simulink model "tp2"  (R2013a)
settings: Solver=ode45  StartTime=0.0  StopTime=0.1  RelTol=1e-3
libraries: powerlib x15, simulink x1
settings Model: Creator=DELL  LastModifiedBy=DELL

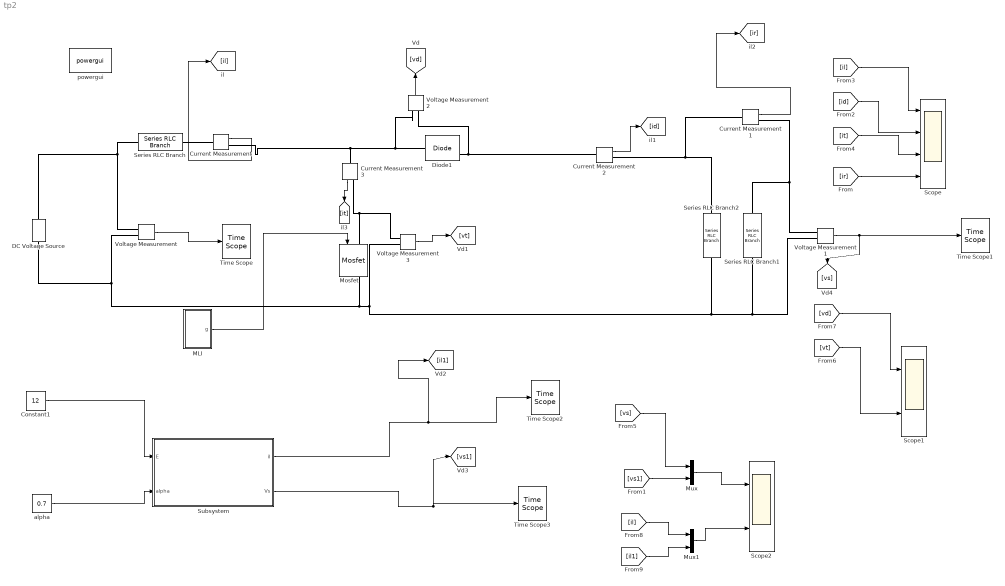
== system tp2 ==
  Constant1 : Constant  Value=12
  Current Measurement{,1..3} (4 alike) : powerlib/Measurements/Current Measurement  PhasorSimulation=off  OutputType=Complex  PSBequivalent=0
  DC Voltage Source : powerlib/Electrical Sources/DC Voltage Source  Amplitude=12  Measurements=Voltage
  Diode1 : powerlib/Power Electronics/Diode  Ron=0.001  Lon=0  Vf=0.8  IC=0  UseSnubber=off  Rs=500  Cs=0  Measurements=on
  "MLI " : Subsystem
  Mosfet : powerlib/Power Electronics/Mosfet  Ron=0.1  Lon=0  Rd=0.01  Vfd=0  IC=0  Rs=1e5  Cs=inf  Measurements=on
  Mux : Mux  Inputs=2
  Mux1 : Mux  Inputs=2
  Scope : Scope  NumInputPorts=4
      settings: YMin=-5~-5~-5~-5  YMax=5~5~5~5
  Scope1 : Scope  NumInputPorts=2
      settings: YMin=-5~-5  YMax=5~5
  Scope2 : Scope  NumInputPorts=2
      settings: YMin=-5~-5  YMax=5~5  SaveName=ScopeData2
  Series RLC Branch : powerlib/Elements/Series RLC Branch  LConnTagsString=__new0  RConnTagsString=__new0  BranchType=L  Resistance=1  Inductance=76.8e-6  SetiL0=off  InitialCurrent=0  Capacitance=1e-6  Setx0=off  InitialVoltage=0  Measurements=None
  Series RLC Branch1 : powerlib/Elements/Series RLC Branch  LConnTagsString=__new0  RConnTagsString=__new0  BranchType=R  Resistance=4  Inductance=1e-3  SetiL0=off  InitialCurrent=0  Capacitance=1e-6  Setx0=off  InitialVoltage=0  Measurements=None
  Series RLC Branch2 : powerlib/Elements/Series RLC Branch  LConnTagsString=__new0  RConnTagsString=__new0  BranchType=C  Resistance=1  Inductance=1e-3  SetiL0=off  InitialCurrent=0  Capacitance=400e-6  Setx0=off  InitialVoltage=0  Measurements=None
  Subsystem : Subsystem
  Time Scope{,1..3} (4 alike) : TimeScope  DefaultConfigurationName=spbscopes.TimeScopeBlockCfg
      settings: CopyFcn=scopeextensions.ScopeBlock.callback(gcbh, 'onBlockCopy', gcbh);  DeleteFcn=scopeextensions.ScopeBlock.callback(gcbh, 'onBlockDelete');  PreSaveFcn=scopeextensions.ScopeBlock.callback(gcbh, 'onModelSave');  NameChangeFcn=scopeextensions.ScopeBlock.callback(gcbh, 'onBlockRename');  CloseFcn=scopeextensions.ScopeBlock.callback(gcbh, 'onBlockClose');  PreDeleteFcn=scopeextensions.ScopeBlock.callback(gcbh, 'onBlockPreDelete');
  Voltage Measurement{,1..3} (4 alike) : powerlib/Measurements/Voltage Measurement  PhasorSimulation=off  OutputType=Complex  PSBequivalent=0
  "alpha " : Constant  Value=0.7
  powergui : powerlib/powergui  Priority=1  SimulationMode=Continuous  SolverType=Tustin  SampleTime=50e-6  frequency=60  SPID=off  DisableSnubberDevices=off  DisableRonSwitches=off  DisableVfSwitches=off  SwTol=0  Interpol=off  DisplayEquations=off  frequencyindice=0  Pbase=100e6  ErrMax=1e-4  Iterations=50  UnitsV=kV  UnitsW=MW  FunctionMessages=off  echomessages=off  HookPort=off  EnableUseOfTLC=off  x0status=blocks  RestoreLinks=warning  ResistiveCurrentMeasurement=off  Frange=[0:2:500]  Ylog=off  Xlog=on  ShowGrid=off  save=off  variable=ZData  ZoomFFT=off  StartTime=0.0  cycles=1  DisplayStyle=1  fundamental=60  FreqAxis=off  MaxFrequency=1000  frequencyindicesteady=1  RmsSteady=1  display=off  Ts=0  methode=off
  wires:
  Voltage Measurement1/1 -> [vs], Time Scope1/1
  Voltage Measurement/1 -> Time Scope/1
  "MLI "/1(g) -> Mosfet/1
  Current Measurement/1 -> [il]
  Voltage Measurement2/1 -> [vd]
  Voltage Measurement3/1 -> [vt]
  [il] -> Scope/1
  [id] -> Scope/2
  [ir] -> Scope/4
  Current Measurement2/1 -> [id]
  Current Measurement1/1 -> [ir]
  [it] -> Scope/3
  Current Measurement3/1 -> [it]
  [vd] -> Scope1/1
  [vt] -> Scope1/2
  Subsystem/1(il) -> [il1], Time Scope2/1
  Constant1/1 -> Subsystem/1(E)
  "alpha "/1 -> Subsystem/2("alpha ")
  Mux/1 -> Scope2/1
  Mux1/1 -> Scope2/2
  Subsystem/2(Vs) -> [vs1], Time Scope3/1
  [vs] -> Mux/1
  [vs1] -> Mux/2
  [il] -> Mux1/1
  [il1] -> Mux1/2
  connections:
  DC Voltage Source/RConn1 -- Voltage Measurement/LConn1 -- Series RLC Branch/LConn1
  DC Voltage Source/LConn1 -- Voltage Measurement/LConn2 -- Mosfet/RConn1 -- Voltage Measurement3/LConn2 -- Series RLC Branch2/RConn1 -- Series RLC Branch1/RConn1 -- Voltage Measurement1/LConn2
  Current Measurement/RConn1 -- Voltage Measurement2/LConn1 -- Diode1/LConn1 -- Current Measurement3/LConn1
  Voltage Measurement2/LConn2 -- Current Measurement2/LConn1 -- Diode1/RConn1
  Series RLC Branch/RConn1 -- Current Measurement/LConn1
  Series RLC Branch1/LConn1 -- Current Measurement1/RConn1 -- Voltage Measurement1/LConn1
  Current Measurement2/RConn1 -- Current Measurement1/LConn1 -- Series RLC Branch2/LConn1
  Voltage Measurement3/LConn1 -- Current Measurement3/RConn1 -- Mosfet/LConn1

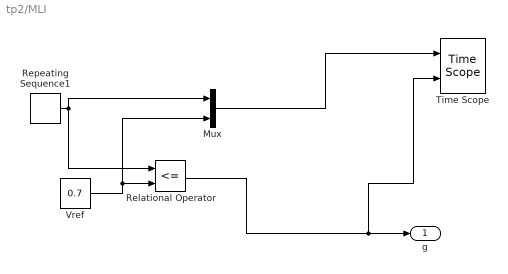
== system tp2/MLI  ==
  Mux : Mux  Inputs=2
  Relational Operator : RelationalOperator  Operator=<=  OutDataTypeStr=boolean
  Repeating Sequence1 : simulink/Sources/Repeating Sequence  rep_seq_t=[0 (1/20000) (1/10000)]  rep_seq_y=[0 1 0]
  Time Scope : TimeScope  NumInputPorts=2  DefaultConfigurationName=spbscopes.TimeScopeBlockCfg
      settings: CopyFcn=scopeextensions.ScopeBlock.callback(gcbh, 'onBlockCopy', gcbh);  DeleteFcn=scopeextensions.ScopeBlock.callback(gcbh, 'onBlockDelete');  PreSaveFcn=scopeextensions.ScopeBlock.callback(gcbh, 'onModelSave');  NameChangeFcn=scopeextensions.ScopeBlock.callback(gcbh, 'onBlockRename');  CloseFcn=scopeextensions.ScopeBlock.callback(gcbh, 'onBlockClose');  PreDeleteFcn=scopeextensions.ScopeBlock.callback(gcbh, 'onBlockPreDelete');
  Vref : Constant  Value=0.7
  g : Outport
  wires:
  Vref/1 -> Relational Operator/2, Mux/2
  Relational Operator/1 -> g/1, Time Scope/2
  Mux/1 -> Time Scope/1
  Repeating Sequence1/1 -> Mux/1, Relational Operator/1

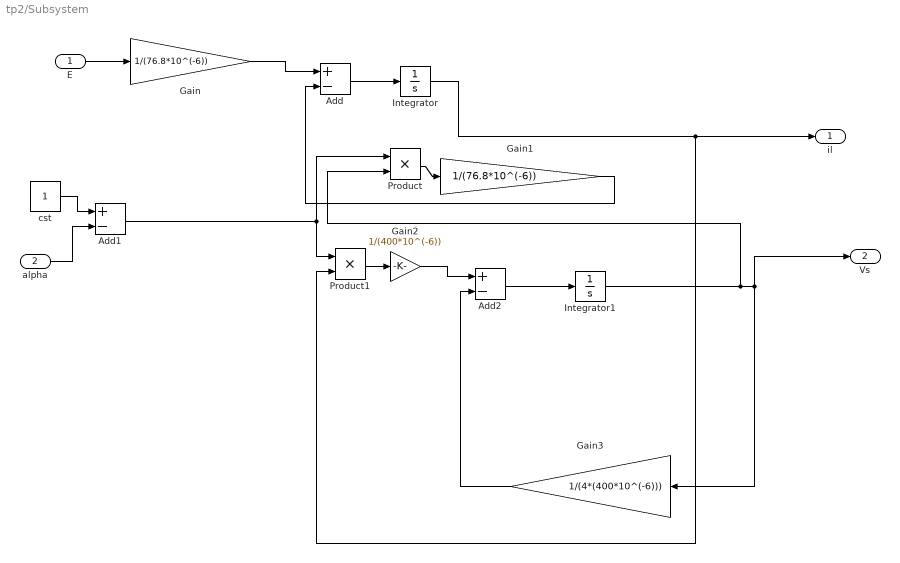
== system tp2/Subsystem ==
  E : Inport
  "alpha " : Inport  Port=2
  Add : Sum  Inputs=+-
  Add1 : Sum  Inputs=+-
  Add2 : Sum  Inputs=+-
  Gain : Gain  Gain=1/(76.8*10^(-6))
  Gain1 : Gain  Gain=1/(76.8*10^(-6))
  Gain2 : Gain  Gain=1/(400*10^(-6))
  Gain3 : Gain  Gain=1/(4*(400*10^(-6)))
  Integrator : Integrator
  Integrator1 : Integrator
  Product : Product
  Product1 : Product
  "cst " : Constant
  il : Outport
  Vs : Outport  Port=2
  wires:
  Add2/1 -> Integrator1/1
  Gain2/1 -> Add2/1
  Gain3/1 -> Add2/2
  E/1 -> Gain/1
  Add1/1 -> Product/1, Product1/1
  Add/1 -> Integrator/1
  Gain1/1 -> Add/2
  "cst "/1 -> Add1/1
  Gain/1 -> Add/1
  Product/1 -> Gain1/1
  Integrator/1 -> il/1, Product1/2
  Product1/1 -> Gain2/1
  Integrator1/1 -> Product/2, Vs/1, Gain3/1
  "alpha "/1 -> Add1/2
